simulink model "tutorial04_second_order"  (R2025a)
settings: Solver=VariableStepAuto  StartTime=0.0  StopTime=10.0  RelTol=1e-3
settings Model: Creator=xing2  LastModifiedBy=xing2

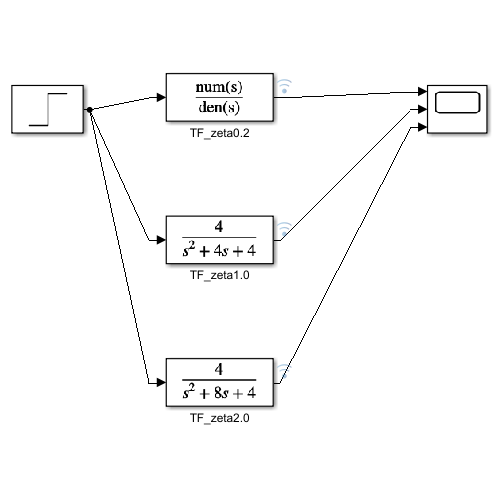
[thumbnail: Simulink's stored preview of the top-level diagram]
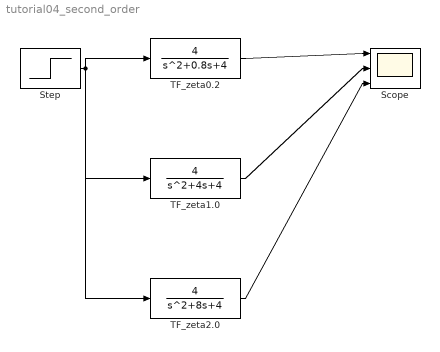
== system tutorial04_second_order ==
  Scope : Scope  NumInputPorts=3
  Step : Step  SampleTime=0
  TF_zeta0.2 : TransferFcn  Numerator=4  Denominator=[1 0.8 4]
  TF_zeta1.0 : TransferFcn  Numerator=4  Denominator=[1 4 4]
  TF_zeta2.0 : TransferFcn  Numerator=4  Denominator=[1 8 4]
  wires:
  Step/1 -> TF_zeta0.2/1, TF_zeta1.0/1, TF_zeta2.0/1
  TF_zeta0.2/1 -> Scope/1
  TF_zeta1.0/1 -> Scope/2
  TF_zeta2.0/1 -> Scope/3
